simulink model "clarkD"  (R2018a)
settings: Solver=ode23tb  StartTime=0.0  StopTime=0.015  RelTol=1e-3
PreLoadFcn:
  | l1=50;
libraries: powerlib x8, powerlib_meascontrol x4, dspswit3 x3, dspsigops x3, simulink x2
(part 2 of 2)

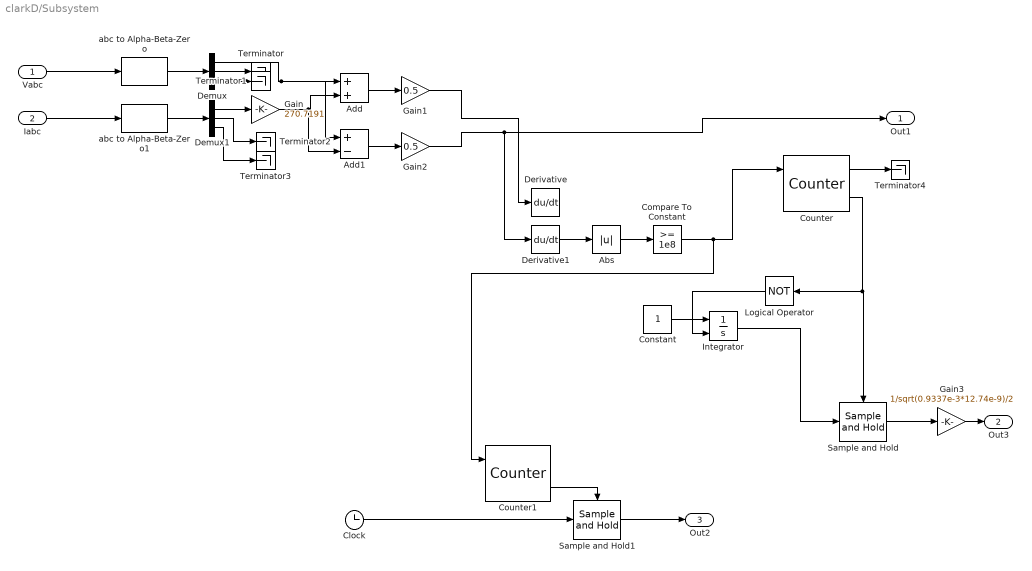
== system clarkD/Subsystem ==
  Vabc : Inport
  Iabc : Inport  Port=2
  Abs : Abs
  Add : Sum
  Add1 : Sum  Inputs=+-
  Clock : Clock
  Compare To Constant : simulink/Logic and Bit Operations/Compare To Constant  relop=>=  const=1e8  OutDataTypeStr=boolean
  Constant : Constant
  Counter : dspswit3/Counter  Direction=Up  CountEvent=Rising edge  CounterSize=User defined  MaxCount=1024  InitialCount=0  Output=Count and Hit  HitValue=2  ResetInput=on  SamplesPerFrame=1  Ts=1  CntDtype=double  HitDtype=Logical
  Counter1 : dspswit3/Counter  Direction=Up  CountEvent=Rising edge  CounterSize=User defined  MaxCount=1024  InitialCount=0  Output=Count and Hit  HitValue=1  ResetInput=on  SamplesPerFrame=1  Ts=1  CntDtype=double  HitDtype=Logical
  Demux : Demux  Outputs=3
  Demux1 : Demux  Outputs=3
  Derivative : Derivative
  Derivative1 : Derivative
  Gain : Gain  Gain=270.7191
  Gain1 : Gain  Gain=0.5
  Gain2 : Gain  Gain=0.5
  Gain3 : Gain  Gain=1/sqrt(0.9337e-3*12.74e-9)/2
  Integrator : Integrator  ExternalReset=level hold
  Logical Operator : Logic  Operator=NOT  AllPortsSameDT=off  OutDataTypeStr=boolean
  Sample and Hold : dspsigops/Sample and Hold  trig=Falling edge  initCond=0  latchinput=on
  Sample and Hold1 : dspsigops/Sample and Hold  trig=Rising edge  initCond=0  latchinput=on
  Terminator{,1..4} (5 alike) : Terminator
  abc to Alpha-Beta-Zero : powerlib_meascontrol/Transformations/abc to Alpha-Beta-Zero
      settings: SourceProductName=Simscape Power Systems
  abc to Alpha-Beta-Zero1 : powerlib_meascontrol/Transformations/abc to Alpha-Beta-Zero
      settings: SourceProductName=Simscape Power Systems
  Out1 : Outport
  Out3 : Outport  Port=2
  Out2 : Outport  Port=3
  wires:
  Iabc/1 -> abc to Alpha-Beta-Zero1/1
  Counter/2 -> Sample and Hold/Trigger, Logical Operator/1
  Gain1/1 -> Derivative/1
  Sample and Hold/1 -> Gain3/1
  Demux/2 -> Terminator/1
  Demux/3 -> Terminator1/1
  Logical Operator/1 -> Integrator/2
  Demux1/3 -> Terminator3/1
  Abs/1 -> Compare To Constant/1
  Counter/1 -> Terminator4/1
  abc to Alpha-Beta-Zero1/1 -> Demux1/1
  Demux/1 -> Add1/1, Add/1
  Gain3/1 -> Out3/1
  Integrator/1 -> Sample and Hold/1
  Gain/1 -> Add1/2, Add/2
  abc to Alpha-Beta-Zero/1 -> Demux/1
  Demux1/1 -> Gain/1
  Add1/1 -> Gain2/1
  Add/1 -> Gain1/1
  Demux1/2 -> Terminator2/1
  Derivative1/1 -> Abs/1
  Constant/1 -> Integrator/1
  Vabc/1 -> abc to Alpha-Beta-Zero/1
  Compare To Constant/1 -> Counter1/1, Counter/1
  Clock/1 -> Sample and Hold1/1
  Counter1/2 -> Sample and Hold1/Trigger
  Sample and Hold1/1 -> Out2/1
  Gain2/1 -> Out1/1, Derivative1/1

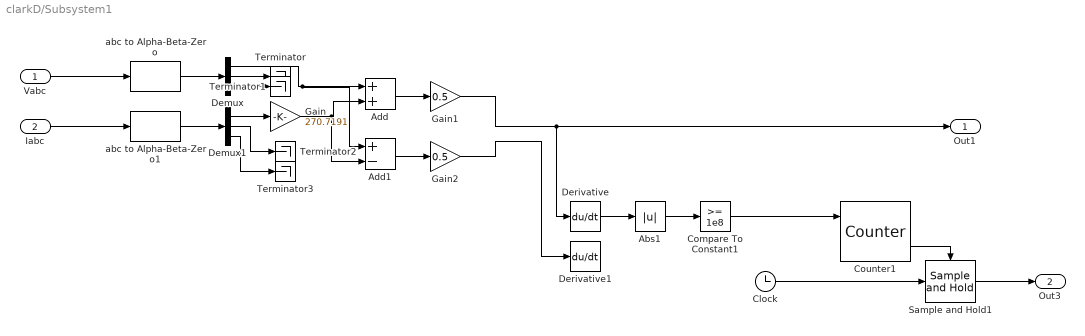
== system clarkD/Subsystem1 ==
  Vabc : Inport
  Iabc : Inport  Port=2
  Abs1 : Abs
  Add : Sum
  Add1 : Sum  Inputs=+-
  Clock : Clock
  Compare To Constant1 : simulink/Logic and Bit Operations/Compare To Constant  relop=>=  const=1e8  OutDataTypeStr=boolean
  Counter1 : dspswit3/Counter  Direction=Up  CountEvent=Rising edge  CounterSize=User defined  MaxCount=1024  InitialCount=0  Output=Count and Hit  HitValue=1  ResetInput=on  SamplesPerFrame=1  Ts=1  CntDtype=double  HitDtype=Logical
  Demux : Demux  Outputs=3
  Demux1 : Demux  Outputs=3
  Derivative : Derivative
  Derivative1 : Derivative
  Gain : Gain  Gain=270.7191
  Gain1 : Gain  Gain=0.5
  Gain2 : Gain  Gain=0.5
  Sample and Hold1 : dspsigops/Sample and Hold  trig=Rising edge  initCond=0  latchinput=on
  Terminator{,1..3} (4 alike) : Terminator
  abc to Alpha-Beta-Zero : powerlib_meascontrol/Transformations/abc to Alpha-Beta-Zero
      settings: SourceProductName=Simscape Power Systems
  abc to Alpha-Beta-Zero1 : powerlib_meascontrol/Transformations/abc to Alpha-Beta-Zero
      settings: SourceProductName=Simscape Power Systems
  Out1 : Outport
  Out3 : Outport  Port=2
  wires:
  Vabc/1 -> abc to Alpha-Beta-Zero/1
  Demux1/2 -> Terminator2/1
  Add/1 -> Gain1/1
  Add1/1 -> Gain2/1
  Demux1/1 -> Gain/1
  abc to Alpha-Beta-Zero/1 -> Demux/1
  Gain/1 -> Add/2, Add1/2
  Gain2/1 -> Derivative1/1
  Demux/1 -> Add/1, Add1/1
  abc to Alpha-Beta-Zero1/1 -> Demux1/1
  Demux1/3 -> Terminator3/1
  Demux/3 -> Terminator1/1
  Demux/2 -> Terminator/1
  Iabc/1 -> abc to Alpha-Beta-Zero1/1
  Clock/1 -> Sample and Hold1/1
  Counter1/2 -> Sample and Hold1/Trigger
  Sample and Hold1/1 -> Out3/1
  Derivative/1 -> Abs1/1
  Abs1/1 -> Compare To Constant1/1
  Compare To Constant1/1 -> Counter1/1
  Gain1/1 -> Out1/1, Derivative/1

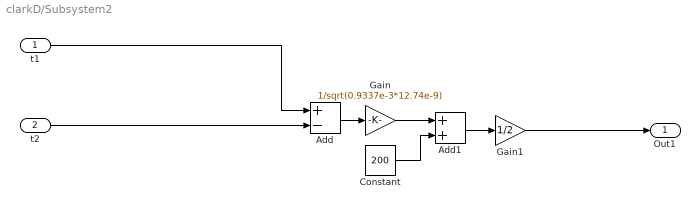
== system clarkD/Subsystem2 ==
  t1 : Inport
  t2 : Inport  Port=2
  Add : Sum  Inputs=+-
  Add1 : Sum
  Constant : Constant  Value=200
  Gain : Gain  Gain=1/sqrt(0.9337e-3*12.74e-9)
  Gain1 : Gain  Gain=1/2
  Out1 : Outport
  wires:
  Constant/1 -> Add1/2
  Add1/1 -> Gain1/1
  Add/1 -> Gain/1
  Gain/1 -> Add1/1
  t2/1 -> Add/2
  Gain1/1 -> Out1/1
  t1/1 -> Add/1
